simulink model "ex3_6"  (R2017a)
settings: Solver=ode23t  StartTime=0.0  StopTime=.2  MaxStep=1e-5  RelTol=1e-3
libraries: powerlib x8, powerlib_meascontrol x1
settings Model: Creator=Omid  LastModifiedBy=Omid
settings SolverCC: ZeroCrossAlgorithm=Adaptive
settings DataIOCC: ReturnWorkspaceOutputs=on
settings DebuggingCC: IgnoredZcDiagnostic=none  UnconnectedInputMsg=none  UnconnectedOutputMsg=none  UnconnectedLineMsg=none
settings SFSimCC: SimUseLocalCustomCode=on
settings RTWCC: RTWUseLocalCustomCode=on

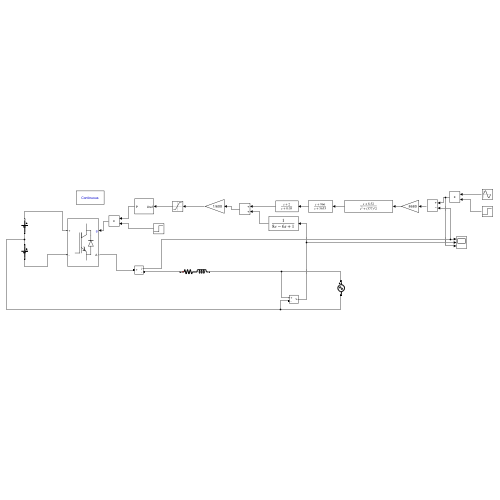
[thumbnail: Simulink's stored preview of the top-level diagram]
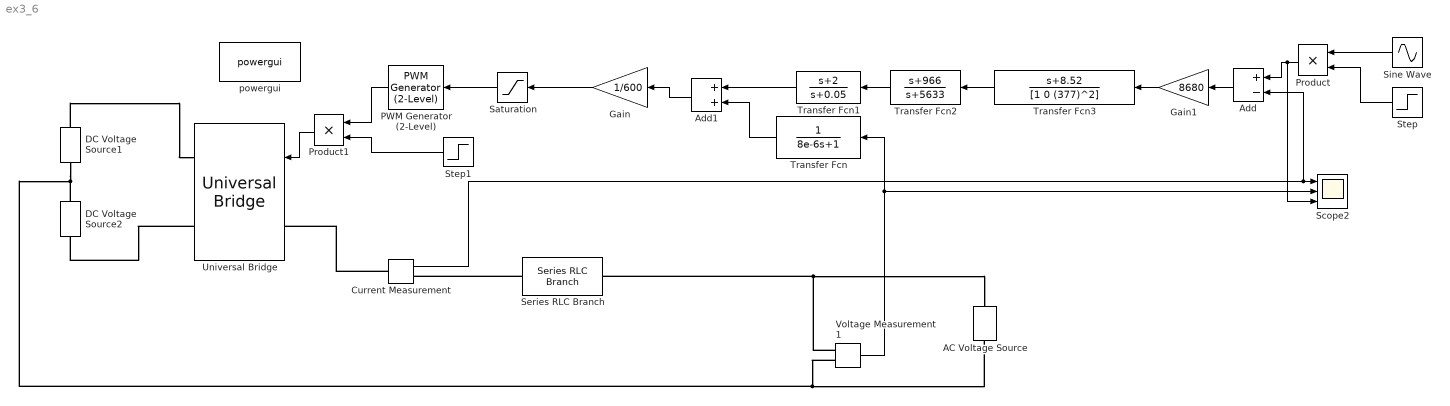
== system ex3_6 ==
  AC Voltage Source : powerlib/Electrical Sources/AC Voltage Source  Amplitude=400  Phase=0  Frequency=60  SampleTime=0  Measurements=None  BusType=swing  Pref=10e3  Qref=0  Qmin=-inf  Qmax=+inf
  Add : Sum  Inputs=+-
  Add1 : Sum
  Current Measurement : powerlib/Measurements/Current Measurement  PhasorSimulation=off  OutputType=Complex  PSBequivalent=0
  DC Voltage Source1 : powerlib/Electrical Sources/DC Voltage Source  Amplitude=600  Measurements=None
  DC Voltage Source2 : powerlib/Electrical Sources/DC Voltage Source  Amplitude=600  Measurements=None
  Gain : Gain  Gain=1/600
  Gain1 : Gain  Gain=8680
  PWM Generator (2-Level) : powerlib_meascontrol/Pulse & Signal Generators/PWM Generator (2-Level)  ModulatorType=Single-phase half-bridge (2 pulses)  ModulatorMode=Unsynchronized  Fc=3420  Pc=90  nF=27  MinMax="[ -1  1 ]"  SamplingTechnique=Natural  ModulatingSignals=off  m=0.8  Freq=60  Phase=0  Ts=0  ShowCarrierOutport=off
  Product : Product
  Product1 : Product
  Saturation : Saturate  UpperLimit=1  LowerLimit=-1
  Scope2 : Scope  NumInputPorts=3
  Series RLC Branch : powerlib/Elements/Series RLC Branch  LConnTagsString=__new0  RConnTagsString=__new0  BranchType=RL  Resistance=.005  Inductance=690e-6  SetiL0=off  InitialCurrent=1600  Capacitance=1e-6  Setx0=off  InitialVoltage=0  Measurements=None
  Sine Wave : Sin  Amplitude=1000  Frequency=2*pi*60  SampleTime=0
  Step : Step  Time=.1  SampleTime=0
  Step1 : Step  Time=.1  SampleTime=0
  Transfer Fcn : TransferFcn  Denominator=[8e-6 1]
  Transfer Fcn1 : TransferFcn  Numerator=[1 2]  Denominator=[1 0.05]
  Transfer Fcn2 : TransferFcn  Numerator=[1 966]  Denominator=[1 5633]
  Transfer Fcn3 : TransferFcn  Numerator=[1 8.52]  Denominator=[1 0 (377)^2]
  Universal Bridge : powerlib/Power Electronics/Universal Bridge  Arms=1  SnubberResistance=1e5  SnubberCapacitance=inf  Device=IGBT / Diodes  Ron=.88e-3  Lon=0  ForwardVoltages="[  1  1 ]"  ForwardVoltage=0  GTOparameters=[ 10e-6 , 20e-6 ]  IGBTparameters=[ 1e-6 , 2e-6 ]  Measurements=None  Measurements_2=None  converterType=Rectifier
  Voltage Measurement1 : powerlib/Measurements/Voltage Measurement  PhasorSimulation=off  OutputType=Complex  PSBequivalent=0
  powergui : powerlib/powergui  Priority=1  SimulationMode=Continuous  SampleTime=50e-6  frequency=60  Iterations=50  frequencyindice=0  Pbase=100e6  ErrMax=1e-4  UnitsV=kV  UnitsW=MW  buscounter=0  FunctionMessages=off  echomessages=off  EnableUseOfTLC=off  CurrentSourceSwitches=off  DisableSnubberDevices=off  DisableRonSwitches=off  DisableVfSwitches=off  DisplayEquations=off  AutomaticDiscreteSolvers=off  SolverType=Tustin/Backward Euler (TBE)  Interpol=off  ExternalGateDelay=off  methode=off  Ts=100  x0status=blocks  SPID=on  SwTol=0  HookPort=off  NonlinearTolerance=1e-4  nMaxIteration=100  ContinueOnMaxIteration=off  RestoreLinks=warning  ResistiveCurrentMeasurement=off  Frange=[0:2:500]  Ylog=off  Xlog=on  ShowGrid=off  save=off  variable=ZData  structure=0  ZoomFFT=off  StartTime=0.0  cycles=1  DisplayStyle=1  fundamental=60  FreqAxis=off  MaxFrequency=1000  frequencyindicesteady=1  RmsSteady=1  display=off
  wires:
  Sine Wave/1 -> Product/1
  Saturation/1 -> PWM Generator (2-Level)/1
  Gain/1 -> Saturation/1
  Add1/1 -> Gain/1
  Current Measurement/1 -> Scope2/1, Add/2
  Voltage Measurement1/1 -> Transfer Fcn/1, Scope2/2
  Transfer Fcn/1 -> Add1/2
  Product/1 -> Scope2/3, Add/1
  Step/1 -> Product/2
  Step1/1 -> Product1/2
  PWM Generator (2-Level)/1 -> Product1/1
  Product1/1 -> Universal Bridge/1
  Transfer Fcn1/1 -> Add1/1
  Add/1 -> Gain1/1
  Transfer Fcn2/1 -> Transfer Fcn1/1
  Transfer Fcn3/1 -> Transfer Fcn2/1
  Gain1/1 -> Transfer Fcn3/1
  connections:
  DC Voltage Source1/RConn1 -- Universal Bridge/RConn1
  Universal Bridge/RConn2 -- DC Voltage Source2/LConn1
  Current Measurement/LConn1 -- Universal Bridge/LConn1
  Series RLC Branch/LConn1 -- Current Measurement/RConn1
  DC Voltage Source2/RConn1 -- AC Voltage Source/LConn1 -- Voltage Measurement1/LConn2 -- DC Voltage Source1/LConn1
  Voltage Measurement1/LConn1 -- Series RLC Branch/RConn1 -- AC Voltage Source/RConn1
